simulink model "parrotMinidroneWaypointFollower"  (R2021b)
settings: Solver=ode3  StartTime=0  StopTime=TFinal  FixedStep=Ts  RelTol=1e-3  EnableMultiTasking=on
undefined symbols (not defined in the file or in its folder): Command, ft, gcbh, init, m, Rec, s, SDTV, sensorCalibrationData, Sensors, sigbuilder_block, States, stop_time, takeOffDuration, Ts, Vehicle, vrmfunc, VTs
libraries: simulink x16, aerolibconvert2 x4, environmentLibrary x2, visionconversions x2, visiongeotforms x2, aerolibutil x2, aerolibanimutils x1, aerolibnav x1, vrlib x1
(part 3 of 3)

== system parrotMinidroneWaypointFollower/Sensors Model/Sensors (Feedthrough)/Sensor System/IMU_Pressure/HAL_acquisition_creator/HAL_ultrasound_SI_creator/HAL_list_echo_t_creator1/HAL_echo_t_creator ==
  Bus Creator6 : BusCreator  Inputs=7  OutDataTypeStr=Bus: HAL_echo_t  NonVirtualBus=on
  begin_echo_index{,1,4,6} (4 alike) : Constant  Value=0  OutDataTypeStr=uint16
  begin_echo_index2 : Constant  Value=0  OutDataTypeStr=int16
  begin_echo_index3 : Constant  Value=0  OutDataTypeStr=int32
  begin_echo_index5 : Constant  Value=0  OutDataTypeStr=int16
  HAL_echo_t : Outport  OutDataTypeStr=Bus: HAL_echo_t  VectorParamsAs1DForOutWhenUnconnected=off
  wires:
  Bus Creator6/1 -> HAL_echo_t/1  "HAL_echo_t"
  begin_echo_index/1 -> Bus Creator6/1  "begin_echo_index"
  begin_echo_index1/1 -> Bus Creator6/2  "end_echo_index"
  begin_echo_index2/1 -> Bus Creator6/3  "max_value_index"
  begin_echo_index3/1 -> Bus Creator6/4  "max_value"
  begin_echo_index4/1 -> Bus Creator6/5  "precedent"
  begin_echo_index5/1 -> Bus Creator6/6  "d_echo"
  begin_echo_index6/1 -> Bus Creator6/7  "pre_max_index"
